simulink library "Pcl812fbk"  (Simulink 4.00)
settings Model: LastModifiedBy=Administrator

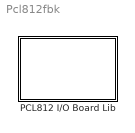
== system Pcl812fbk ==
  PCL812 I/O Board Lib : Subsystem
      settings: RTWFcnNameOpts=Auto  RTWFileNameOpts=Auto
      mask Type: PCL812 I/O Board Lib
      mask Display: plot(0,0,100,100,[90,80,80,11,11],[90,90,20,20,80],[11,80],[80,80],[80,80],[20,14],[80,85,85,80],[45,45,66,66],[45,45,74,74],[20,13,13,20],[15,27,27,15,15],[75,75,26,26,75],[33,48,48,33,33],[75,75,55,55,75],[55,55,71,71,55],[55,75,75,55,55],[33,41,41,33,33],[50,50,27,27,50],[48,56,56,48,48],[50,50,27,27,50],[62,70,70,62,62],[50,50,27,27,50])

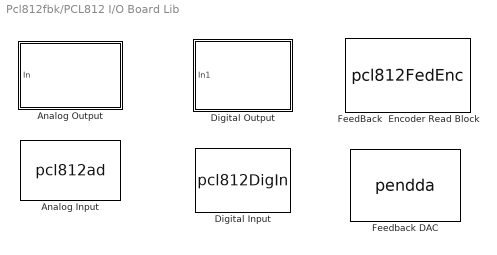
== system Pcl812fbk/PCL812 I/O Board Lib ==
  Analog Input : S-Function  FunctionName=pcl812ad  Parameters=baseAddr, inputChannel, AdcGain, AdcRange, stime,hwAcces  PortCounts=[]  SFunctionModules=''  mask(Analog Output Module){baseAddr=0x220, inputChannel=0, AdcGain=1, AdcRange=5, stime=0.001, hwAcces=on}
      mask prompts: baseAddr "Base I/O Address :"; inputChannel "Input Channel :"; AdcGain "ADC Gain (1, 2, 4, 8, 16)"; AdcRange "ADC Range (either 5 or 10)"; stime "Sample Time (sec):"; hwAcces "Access Hardware"
      mask Display: disp('PCL812PG\n Lab I/O Board \n\n ADC')
  Analog Output : Subsystem  mask(Analog Output Module){baseAddr=0x220, outChannel=0, dacRef=5.0, stime=0.001, hwAcces=on}
      mask prompts: baseAddr "Base I/O Address:"; outChannel "Output Channel"; dacRef "Dac Reference Voltage"; stime "sample Time (sec):"; hwAcces "Access Hardware"
      mask help: Digital to Analog Output block for the PCL812 I/O board
      settings: RTWFcnNameOpts=Auto  RTWFileNameOpts=Auto
      mask Help: no help is given for this block
      mask Display: disp('PCL812PG\n Lab I/O Board \n\n DAC')
  Digital Input : S-Function  FunctionName=pcl812DigIn  Parameters='0x220',0, 0.001, 1  PortCounts=[]  SFunctionModules=''  mask(Digital Input Module){baseAddr=0x220, InByte=0, stime=0.001, hwAcces=on}
      mask prompts: baseAddr "Base I/O Address :"; InByte "Input Byte ('0' for Low '1' for High Byte)"; stime "Sample Time (sec)"; hwAcces "Acces Hardware"
      mask Display: disp('PCL812PG\n Lab I/O Board \n\n Digital Input')
  Digital Output : Subsystem  mask(Digital Output Model){baseAddr=0x220, outByte=0, stime=0.001, hwAcces=on}
      mask prompts: baseAddr "Base I/O Address:"; outByte "Output Byte ('0' for Low '1'  for High Byte)"; stime "Sample Time (sec):"; hwAcces "Acces Hardware"
      settings: RTWFcnNameOpts=Auto  RTWFileNameOpts=Auto
      mask Display: disp('PCL812PG\n Lab I/O Board \n\n Digital Output')
  FeedBack  Encoder Read Block : S-Function  FunctionName=pcl812FedEnc  Parameters=baseAddr, Channel, stime ,encOffSet,hwAcces  PortCounts=[]  SFunctionModules=''  mask(Encoder Module for FeedBack Experiments){baseAddr=0x220, Channel=1, stime=0.001, encOffSet=0, hwAcces=on}
      mask prompts: baseAddr "Base I/O Address :"; Channel "Channel (either 0 or 1)"; stime "sampling Time (sec) :"; encOffSet "Encoder Offset"; hwAcces "Access Hardware"
      mask help: Special block to use with the Feedback Experiments to read encoder signals using the digital IO lines
      mask Display: disp('PCL812PG\n Lab I/O Board \n\n FeedBackEncoder')
  Feedback DAC : S-Function  FunctionName=pendda  Parameters=baseAddr,outChannel, dacRef, stime, hwAcces  PortCounts=[]  SFunctionModules=''  mask(DAC for Feebback Experiments){baseAddr=0x220, outChannel=1, dacRef=5, stime=0.001, hwAcces=on}
      mask prompts: baseAddr "Base I/O Address :"; outChannel "Output Channel"; dacRef "Dac Reference Voltage"; stime "Sample Time (sec):"; hwAcces "Access Hardware"
      mask Display: disp('PCL812PG\n Lab I/O Board \n\n FeedBack  DAC')

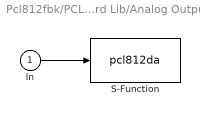
== system Pcl812fbk/PCL812 I/O Board Lib/Analog Output ==
  In : Inport  Port=1
  S-Function : S-Function  FunctionName=pcl812da  Parameters=baseAddr,outChannel, dacRef, stime, hwAcces  PortCounts=[]  SFunctionModules=''
  wires:
  In/1 -> S-Function/1

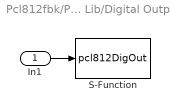
== system Pcl812fbk/PCL812 I/O Board Lib/Digital Output ==
  In1 : Inport  Port=1
  S-Function : S-Function  FunctionName=pcl812DigOut  Parameters=baseAddr,outByte, stime, hwAcces  PortCounts=[]  SFunctionModules=''
  wires:
  In1/1 -> S-Function/1
